simulink model "motorsim"  (R2015b)
settings: Solver=ode4  StartTime=0.0  StopTime=2  FixedStep=0.001  RelTol=1e-3
values from neighbouring files (symbols this model uses):
  alpha = 1/K(1)    [lsrl.m]    (also in parameters.m = 66.9379)
  Kd = (2*zeta*omega+p-tau)/alpha    [parameters.m]
  Kg = 70    [parameters.m]
  Ki = (omega^2*p)/alpha    [parameters.m]
  Kp = (omega^2+2*zeta*omega*p)/alpha    [parameters.m]
  tau = alpha*K(2)    [lsrl.m]    (also in parameters.m = 39.3285)
undefined symbols (not defined in the file or in its folder): qc_get_step_size
libraries: quarc_library x4, simulink x1
settings Model: SimulationMode=external  ExtModeTrigDuration=10000  ExtModeArchiveMode=auto  ExtModeArchiveFileName=data.mat  ExtModeArchiveDirName=U:\ECE433\lab4  Creator=millerid  LastModifiedBy=flynng
settings SolverCC: PositivePriorityOrder=on
settings RTWCC: SystemTargetFile=quarc_win64.tlc  TemplateMakefile=quarc_default_tmf  Description=QUARC Win64 Target
settings STFCustomTargetCC: TargetPreCompLibLocation=C:\ProgramData\QUARC\lib\2015b\win64\release  GeneratePreprocessorConditionals=Use local settings  CPPClassGenCompliant=off
settings GRTTargetCC: TargetPreCompLibLocation=C:\ProgramData\QUARC\lib\2015b\win64\release  ParMdlRefBuildCompliant=off  CompOptLevelCompliant=off  CombineOutputUpdateFcns=off  MatFileLogging=off  CPPClassGenCompliant=off  GRTInterface=on  UseToolchainInfoCompliant=off  ExtMode=on  ExtModeMexFile=quarc_comm

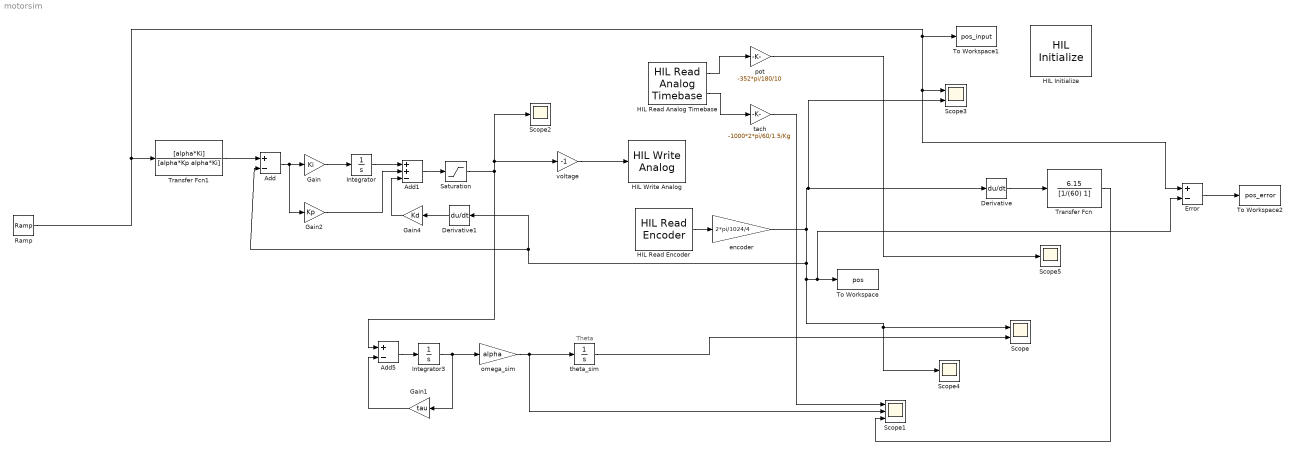
== system motorsim ==
  note: Theta
  Add : Sum  Inputs=+-
  Add1 : Sum  Inputs=++-
  Add5 : Sum  Inputs=+-
  Derivative : Derivative
  Derivative1 : Derivative
  Error : Sum  Inputs=+-
  Gain : Gain  Gain=Ki
  Gain1 : Gain  Gain=tau
  Gain2 : Gain  Gain=Kp
  Gain4 : Gain  Gain=Kd
  HIL Initialize : quarc_library/Data Acquisition/Generic/Configuration/HIL Initialize  Priority=-99  object_name=controller  board_type=q8_usb  board_number=0  board_options=update_rate=normal;decimation=1  exclusive=off  active=off  hardware_clocks=[0:2]  clock_modes=[]  initial_clock_frequencies=[]  set_clock_params_at_start=off  set_clock_params_at_switch_in=off  set_clock_frequencies_at_start=off  set_clock_frequencies_at_switch_in=off  analog_input_channels=[0:7]  analog_input_maximums=10  analog_input_minimums=-10  set_analog_input_params_at_start=on  set_analog_input_params_at_switch_in=off  analog_output_channels=[0:7]  analog_output_maximums=10  analog_output_minimums=-10  initial_analog_outputs=[0]  final_analog_outputs=[0]  watchdog_analog_outputs=0  set_analog_output_params_at_start=on  set_analog_output_params_at_switch_in=off  set_analog_outputs_at_start=on  set_analog_outputs_at_switch_in=off  set_analog_outputs_at_terminate=on  set_analog_outputs_at_switch_out=off  set_analog_outputs_on_watchdog=off  digital_input_channels=[]  digital_output_channels=[]  digital_output_configuration=[]  initial_digital_outputs=[1]  final_digital_outputs=[1]  watchdog_digital_outputs=[1]  set_digital_output_params_at_start=off  set_digital_output_params_at_switch_in=off  set_digital_outputs_at_start=on  set_digital_outputs_at_switch_in=off  set_digital_outputs_at_terminate=on  set_digital_outputs_at_switch_out=off  set_digital_outputs_on_watchdog=off  encoder_channels=[0:7]  quadrature=[4]  encoder_filter_frequency=[]  initial_encoder_counts=[0]  set_encoder_params_at_start=on  set_encoder_params_at_switch_in=off  set_encoder_counts_at_start=on  set_encoder_counts_at_switch_in=off  pwm_channels=[0:7]  pwm_modes=0  pwm_frequency=99.532799999999995e6/4095  pwm_configuration=[0]  pwm_alignment=[0]  pwm_polarity=[1]  pwm_leading_deadband=[0]  pwm_trailing_deadband=[0]  initial_pwm_outputs=[0]  final_pwm_outputs=[0]  watchdog_pwm_outputs=[0]  set_pwm_params_at_start=on  set_pwm_params_at_switch_in=off  set_pwm_outputs_at_start=on  set_pwm_outputs_at_switch_in=off  set_pwm_outputs_at_terminate=on  set_pwm_outputs_at_switch_out=off  set_pwm_outputs_on_watchdog=off  other_output_channels=[]  initial_other_outputs=[]  final_other_outputs=[]  watchdog_other_outputs=[]  set_other_outputs_at_start=off  set_other_outputs_at_switch_in=off  set_other_outputs_at_terminate=off  set_other_outputs_at_switch_out=off  set_other_outputs_on_watchdog=off
  HIL Read Analog Timebase : quarc_library/Data Acquisition/Generic/Timebases/HIL Read Analog Timebase  object_name=controller  clock=0  channels=[0:1]  samples_in_buffer=max(ceil(1/qc_get_step_size), 1)  active=on  vector_output=off
      settings: AttributesFormatString=(%<object_name>)
  HIL Read Encoder : quarc_library/Data Acquisition/Generic/Immediate I//O/HIL Read Encoder  object_name=controller  channels=0  sample_time=qc_get_step_size  active=on  vector_output=off  data_type_mode=Inherit via back propagation  data_type=double
  HIL Write Analog : quarc_library/Data Acquisition/Generic/Immediate I//O/HIL Write Analog  object_name=controller  channels=0  sample_time=-1  active=off  vector_input=off
  Integrator : Integrator
  Integrator3 : Integrator
  Ramp : simulink/Sources/Ramp  slope=pi/2  start=0  X0=0
  Saturation : Saturate  UpperLimit=10  LowerLimit=-10
  Scope : Scope  NumInputPorts=2
  Scope1 : Scope  NumInputPorts=3
  Scope2 : Scope
  Scope3 : Scope  NumInputPorts=2
  Scope4 : Scope
  Scope5 : Scope
  To Workspace : ToWorkspace  VariableName=pos  SampleTime=-1
  To Workspace1 : ToWorkspace  VariableName=pos_input  SampleTime=-1
  To Workspace2 : ToWorkspace  VariableName=pos_error  SampleTime=-1
  Transfer Fcn : TransferFcn  Numerator=[6.15]  Denominator=[1/(60) 1]
  Transfer Fcn1 : TransferFcn  Numerator=[alpha*Ki]  Denominator=[alpha*Kp alpha*Ki]
  encoder : Gain  Gain=2*pi/1024/4
  omega_sim : Gain  Gain=alpha
  pot : Gain  Gain=-352*pi/180/10
  tach : Gain  Gain=-1000*2*pi/60/1.5/Kg
  theta_sim : Integrator
  voltage : Gain  Gain=-1
  wires:
  HIL Read Encoder/1 -> encoder/1
  HIL Read Analog Timebase/1 -> pot/1
  HIL Read Analog Timebase/2 -> tach/1
  omega_sim/1 -> theta_sim/1, Scope1/2
  theta_sim/1 -> Scope/2
  pot/1 -> Scope5/1
  tach/1 -> Scope1/1
  encoder/1 -> Scope3/2, Derivative/1, Error/2, To Workspace/1, Scope/1, Scope4/1, Add/2, Derivative1/1
  voltage/1 -> HIL Write Analog/1
  Integrator3/1 -> omega_sim/1, Gain1/1
  Gain1/1 -> Add5/2
  Add5/1 -> Integrator3/1
  Derivative/1 -> Transfer Fcn/1
  Transfer Fcn/1 -> Scope1/3
  Add1/1 -> Saturation/1
  Derivative1/1 -> Gain4/1
  Gain4/1 -> Add1/3
  Add/1 -> Gain2/1, Gain/1
  Gain/1 -> Integrator/1
  Gain2/1 -> Add1/2
  Integrator/1 -> Add1/1
  Transfer Fcn1/1 -> Add/1
  Ramp/1 -> To Workspace1/1, Error/1, Scope3/1, Transfer Fcn1/1
  Saturation/1 -> voltage/1, Scope2/1, Add5/1
  Error/1 -> To Workspace2/1
